simulink library "Thesis_Sublibraries"  (R2020a)
settings: Solver=VariableStepAuto  StartTime=0.0  StopTime=10.0  RelTol=1e-3
undefined symbols (not defined in the file): cga_Horiz_Param, cgb_Horiz_Param, lead_veh_acc, T_mode, Traffic, V2V_FLAG
libraries: simulink x1
settings Model: Creator=John Jr  LastModifiedBy=John Jr
settings SFSimCC: CustomCodeUndefinedFunction=UseInterfaceOnly

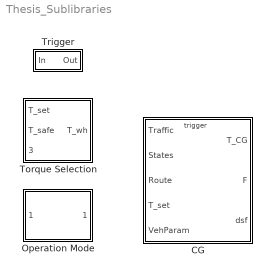
== system Thesis_Sublibraries ==
  CG : Subsystem  TreatAsAtomicUnit=on
      mask Display:
      | patch([0 1 1 0], [0 0 1 1],[.8 1 1])
      | 
      | port_label('input',1,'Traffic')
      | port_label('input',2,'States')
      | port_label('input',3,'Route')
      | port_label('input',4,'T_set')
      | port_label('input',5,'VehParam')
      | 
      | 
      | port_label('output',1,'T_{CG}','texmode','on')
      | port_label('output',2,'F','texmode','on')
      | port_label('output',3,'dsf','texmode','on')
      | 
      | port_label('trigger','\spadesuit','texmode','on')
  Operation Mode : Subsystem  mask{ds_max=200}
      mask prompts: ds_max "Radar Range [m]"
      mask DialogControl Control3 Prompt: Traffic Parameters
      mask Display:
      | patch([0 1 1 0], [0 0 1 1],[.8 1 1])
      | 
      | port_label('input',1,'Traffic')
      | 
      | port_label('output',1,'Mode')
  Torque Selection : Subsystem
      mask Display:
      | patch([0 1 1 0], [0 0 1 1],[.8 1 1])
      | 
      | port_label('input',1,'T_{MPC}','texmode','on')
      | port_label('input',2,'T_{ACC}','texmode','on')
      | port_label('input',3,'Mode')
      | 
      | port_label('output',1,'T_{set}','texmode','on')
  Trigger : Subsystem  mask{f=1}
      mask prompts: f "Trigger Frequency [Hz]"
      mask Display:
      | patch([0 1 1 0], [0 0 1 1],[.8 1 1])
      | 
      | %port_label('input',1,'In')
      | 
      | %port_label('output',1,'Out')
      | 
      | str_f = get_param(gcb,'f');
      | disp(['{\fontname{Cambria Math}f = ' str_f ' Hz}'],'texmode','on')

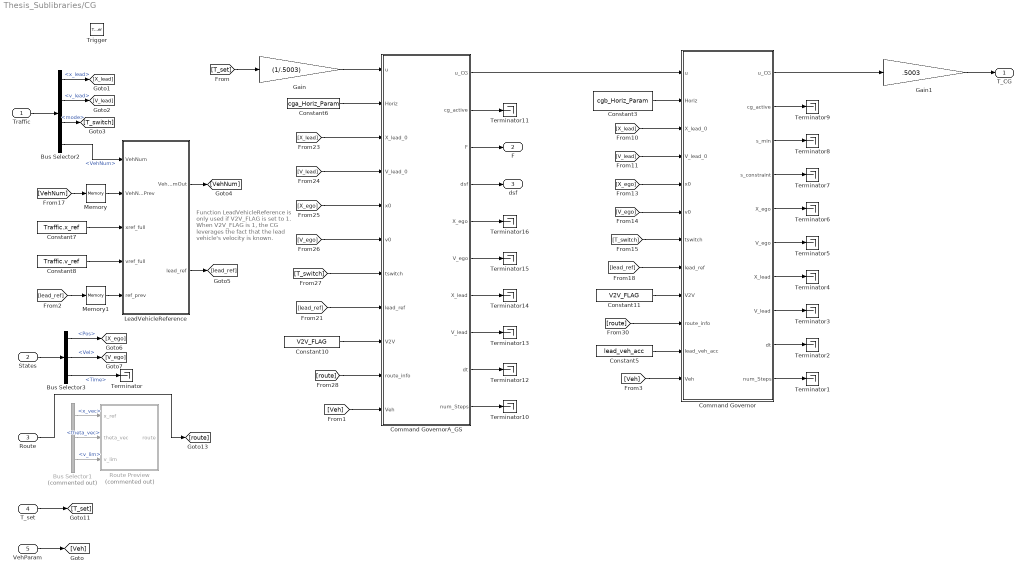
== system Thesis_Sublibraries/CG ==
  note: Function LeadVehicleReference is only used if V2V_FLAG is set to 1. When V2V_FLAG is 1, the CG leverages the fact that the lead vehicle's velocity is known.
  Traffic : Inport
  States : Inport  Port=2
  Route : Inport  Port=3
  T_set : Inport  Port=4
  VehParam : Inport  Port=5
  Trigger : TriggerPort  VariantControl=Variant  PortDimensions=1
  Bus Selector1 : BusSelector  Commented=on  OutputSignals=x_vec,theta_vec,v_lim
  Bus Selector2 : BusSelector  OutputSignals=x_lead,v_lead,mode,VehNum
  Bus Selector3 : BusSelector  OutputSignals=Pos,Vel,Time
  Command Governor : MATLAB Function  TreatAsAtomicUnit=on
  Command GovernorA_GS : MATLAB Function  TreatAsAtomicUnit=on
  Constant10 : Constant  Value=V2V_FLAG
  Constant11 : Constant  Value=V2V_FLAG
  Constant3 : Constant  Value=cgb_Horiz_Param
  Constant5 : Constant  Value=lead_veh_acc
  Constant6 : Constant  Value=cga_Horiz_Param
  Constant7 : Constant  Value=Traffic.x_ref
  Constant8 : Constant  Value=Traffic.v_ref
  Gain : Gain  Gain=(1/.5003)
  Gain1 : Gain  Gain=.5003
  LeadVehicleReference : MATLAB Function  TreatAsAtomicUnit=on
  Memory : Memory  InheritSampleTime=on
  Memory1 : Memory  InheritSampleTime=on
  Route Preview : MATLAB Function  Commented=on  TreatAsAtomicUnit=on
  Terminator{,1..16} (17 alike) : Terminator
  T_CG : Outport  VectorParamsAs1DForOutWhenUnconnected=off
  F : Outport  Port=2  VectorParamsAs1DForOutWhenUnconnected=off
  dsf : Outport  Port=3  VectorParamsAs1DForOutWhenUnconnected=off
  wires:
  Route/1 -> [route]
  Bus Selector3/3 -> Terminator/1  "<Time>"
  Gain1/1 -> T_CG/1
  T_set/1 -> [T_set]
  Bus Selector3/2 -> [V_ego]  "<Vel>"
  Bus Selector3/1 -> [X_ego]  "<Pos>"
  States/1 -> Bus Selector3/1
  Memory/1 -> LeadVehicleReference/2(VehNumPrev)
  [VehNum] -> Memory/1
  Memory1/1 -> LeadVehicleReference/5(ref_prev)
  Constant7/1 -> LeadVehicleReference/3(xref_full)
  LeadVehicleReference/2(lead_ref) -> [lead_ref]
  LeadVehicleReference/1(VehNumOut) -> [VehNum]
  [lead_ref] -> Memory1/1
  Constant8/1 -> LeadVehicleReference/4(vref_full)
  Bus Selector2/4 -> LeadVehicleReference/1(VehNum)  "<VehNum>"
  Bus Selector2/3 -> [T_switch]  "<mode>"
  Bus Selector2/2 -> [V_lead]  "<v_lead>"
  Bus Selector2/1 -> [X_lead]  "<x_lead>"
  Traffic/1 -> Bus Selector2/1
  Bus Selector1/3 -> Route Preview/3(v_lim)  "<v_lim>"
  Bus Selector1/1 -> Route Preview/1(x_ref)  "<x_vec>"
  Bus Selector1/2 -> Route Preview/2(theta_vec)  "<theta_vec>"
  VehParam/1 -> [Veh]
  [T_set] -> Gain/1
  [Veh] -> Command GovernorA_GS/11(Veh)
  Constant11/1 -> Command Governor/9(V2V)
  [Veh] -> Command Governor/12(Veh)
  Command GovernorA_GS/9(dt) -> Terminator12/1
  Command Governor/9(dt) -> Terminator2/1
  [V_lead] -> Command Governor/4(V_lead_0)
  [X_ego] -> Command GovernorA_GS/5(x0)
  [V_ego] -> Command GovernorA_GS/6(v0)
  [T_switch] -> Command Governor/7(tswitch)
  Constant6/1 -> Command GovernorA_GS/2(Horiz)
  Command GovernorA_GS/4(dsf) -> dsf/1
  Command GovernorA_GS/5(X_ego) -> Terminator16/1
  Command GovernorA_GS/1(u_CG) -> Command Governor/1(u)
  [route] -> Command GovernorA_GS/10(route_info)
  Constant10/1 -> Command GovernorA_GS/9(V2V)
  Command Governor/2(cg_active) -> Terminator9/1
  Command Governor/6(V_ego) -> Terminator5/1
  Command GovernorA_GS/2(cg_active) -> Terminator11/1
  [X_lead] -> Command GovernorA_GS/3(X_lead_0)
  [T_switch] -> Command GovernorA_GS/7(tswitch)
  Command GovernorA_GS/7(X_lead) -> Terminator14/1
  Command GovernorA_GS/3(F) -> F/1
  Constant5/1 -> Command Governor/11(lead_veh_acc)
  Command GovernorA_GS/6(V_ego) -> Terminator15/1
  Command Governor/3(s_min) -> Terminator8/1
  [route] -> Command Governor/10(route_info)
  Command GovernorA_GS/10(num_Steps) -> Terminator10/1
  [V_ego] -> Command Governor/6(v0)
  Gain/1 -> Command GovernorA_GS/1(u)
  Command Governor/8(V_lead) -> Terminator3/1
  Command Governor/1(u_CG) -> Gain1/1
  Command Governor/10(num_Steps) -> Terminator1/1
  Constant3/1 -> Command Governor/2(Horiz)
  Command GovernorA_GS/8(V_lead) -> Terminator13/1
  [X_lead] -> Command Governor/3(X_lead_0)
  Command Governor/4(s_constraint) -> Terminator7/1
  Command Governor/7(X_lead) -> Terminator4/1
  [lead_ref] -> Command GovernorA_GS/8(lead_ref)
  Command Governor/5(X_ego) -> Terminator6/1
  [lead_ref] -> Command Governor/8(lead_ref)
  [V_lead] -> Command GovernorA_GS/4(V_lead_0)
  [X_ego] -> Command Governor/5(x0)

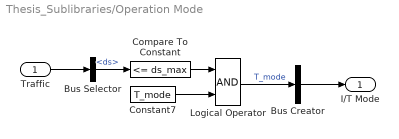
== system Thesis_Sublibraries/Operation Mode ==
  Traffic : Inport
  Bus Creator : BusCreator  Inputs=1
  Bus Selector : BusSelector  OutputSignals=ds
  Compare To Constant : simulink/Logic and Bit Operations/Compare To Constant  relop=<=  const=ds_max  OutDataTypeStr=boolean
  Constant7 : Constant  Value=T_mode
  Logical Operator : Logic  AllPortsSameDT=off  OutDataTypeStr=boolean
  I/T Mode : Outport  VectorParamsAs1DForOutWhenUnconnected=off
  wires:
  Bus Creator/1 -> I/T Mode/1
  Logical Operator/1 -> Bus Creator/1  "T_mode"
  Compare To Constant/1 -> Logical Operator/1
  Bus Selector/1 -> Compare To Constant/1  "<ds>"
  Constant7/1 -> Logical Operator/2
  Traffic/1 -> Bus Selector/1

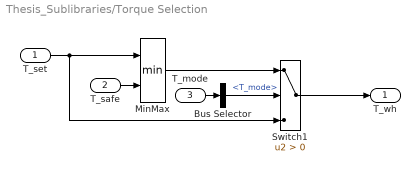
== system Thesis_Sublibraries/Torque Selection ==
  T_set : Inport
  T_safe : Inport  Port=2
  T_mode : Inport  Port=3
  Bus Selector : BusSelector  OutputSignals=T_mode
  MinMax : MinMax  Inputs=2
  Switch1 : Switch  Criteria=u2 > Threshold
  T_wh : Outport  VectorParamsAs1DForOutWhenUnconnected=off
  wires:
  T_safe/1 -> MinMax/2
  T_set/1 -> Switch1/3, MinMax/1
  MinMax/1 -> Switch1/1
  Bus Selector/1 -> Switch1/2  "<T_mode>"
  T_mode/1 -> Bus Selector/1
  Switch1/1 -> T_wh/1

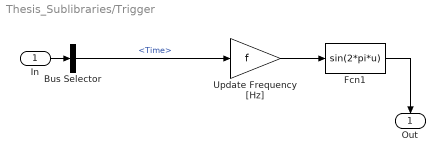
== system Thesis_Sublibraries/Trigger ==
  In : Inport
  Bus Selector : BusSelector  OutputSignals=Time
  Fcn1 : Fcn  Expr=sin(2*pi*u)
  Update Frequency [Hz] : Gain  Gain=f
  Out : Outport  VectorParamsAs1DForOutWhenUnconnected=off
  wires:
  Bus Selector/1 -> Update Frequency [Hz]/1  "<Time>"
  Update Frequency [Hz]/1 -> Fcn1/1
  Fcn1/1 -> Out/1
  In/1 -> Bus Selector/1

== matlab function Thesis_Sublibraries/CG/Command Governor ==
  settings: updateMethod=DISCRETE
  data: u input; u_CG output size=1; Horiz input; X_lead_0 input; V_lead_0 input; cg_active output size=1; x0 input; v0 input; tswitch input; s_min output; lead_ref input size=[8000 3]; s_constraint output; X_ego output; V_ego output; X_lead output; V_lead output; dt output size=1; num_Steps output size=1; V2V input; route_info input; lead_veh_acc input; Veh input
function [u_CG, cg_active, s_min, s_constraint, ...
    X_ego, V_ego, X_lead, V_lead, dt, num_Steps] ... 
    = Command_Governor(u, Horiz, X_lead_0, ... 
        V_lead_0, x0, v0, tswitch,...
        lead_ref, V2V, route_info, lead_veh_acc, Veh)
% s_constraint = NaN(1, 80);
s_constraint    = NaN(1, length(Horiz));
X_ego           = zeros(1, length(Horiz));
V_ego           = zeros(1, length(Horiz));
X_lead          = zeros(1, length(Horiz));
V_lead          = V_lead_0.*ones(1, length(Horiz));
Cs_min          = 10;


cg_Step         = Horiz(1);
% num_Steps       = cg_length/cg_Step;
num_Steps       = length(Horiz);
dt              = cg_Step;
u_brk_max       = -120000;

xref = lead_ref(:,1);
vref = lead_ref(:,2);
tref = lead_ref(:,3);

tsafe = 1;

X_vec = route_info(:,1);                                %   rad - Road grade angle vector
theta_vec = route_info(:,2);                            %   rad - Road grade angle vector


amdego          = -3;  
percBuff        = 1;
X_ego(1)        = x0;
V_ego(1)        = v0;
X_lead(1)       = X_lead_0;
d_u             = 200;

t_cg = zeros(1, length(Horiz)+1);
t_cg(2:end) = cumsum(Horiz);

if tswitch ~= 1
    u_CG = u;
    cg_active = 0;
    s_min = nan;
    MAX_FLAG = 0;
else
    if V2V == 1
        t_shift = interpone(xref, tref, X_lead_0);
        
        for i = 2:length(Horiz)
            X_lead(i) = interpone(tref, xref, t_shift + t_cg(i));
            V_lead(i) = interpone(xref, vref, X_lead(i));
        end
    else
        for i = 2:length(Horiz)
            V_lead(i) = V_lead(i-1) + lead_veh_acc*dt;
            X_lead(i) = X_lead(i-1) + ((V_lead(i) + V_lead(i-1))/2)*dt;
        end
    end
    
    
%     amdlead = a_lead_brk_max;
%     i = 1;
%     tstoplead = abs(V_lead(i)/a_lead_brk_max);
%     
%     if a_lead_brk_max == 0
%         s_min = Cs_min;
%     else
%         tstopego = abs(V_ego(i)/amdego);
%         s_min = max(Cs_min, Cs_min + (V_ego(i)*tstopego - V_lead(i)*tstoplead) ...
%                 + ((amdego/2)*tstopego^2 - (amdlead/2)*tstoplead^2));
% 
%     end
    s_min = max(Cs_min, tsafe*V_lead(1));
    
    MAX_FLAG = 0;
    u_CG = u;
    i = 1;
    while i < num_Steps && MAX_FLAG == 0
        
        % Veh(1)    g
        % Veh(2)    rho
        % Veh(3)    m
        % Veh(4)    Cd
        % Veh(5)    A_ref
        % Veh(6)    Cr
        theta = interp1(X_vec, theta_vec, X_ego(i));
        F_grav = Veh(3)*Veh(1)*sin(theta);
        F_road = Veh(3)*Veh(1)*Veh(6)*cos(theta);
        F_aero = (1/2)*Veh(4)*Veh(2)*Veh(5)*V_ego(i)^2;
        V_ego(i+1) = V_ego(i) + (dt/Veh(3))*(u_CG) - percBuff*(dt/Veh(3))*(F_road + F_aero ...
            + max(0, F_grav)) - (dt/Veh(3))*min(0, F_grav)*(1+(1-percBuff));
        X_ego(i+1) = X_ego(i) + ((V_ego(i) + V_ego(i+1))/2)*dt;  
       
        s = X_lead(i) - X_ego(i);
        
%         rho = V_ego(i) - V_lead(i);
%         tstopego = abs(V_ego(i)/amdego);
%         tstoplead = abs(V_lead(i)/a_lead_brk_max);
%         if a_lead_brk_max == 0
%             s_constraint(i) = Cs_min;
%         else
%             
%             s_constraint(i) = max(Cs_min, Cs_min + (V_ego(i)*tstopego ...
%                 - V_lead(i)*tstoplead) ... 
%                 + ((amdego/2)*tstopego^2 - (amdlead/2)*tstoplead^2));
%         end
        s_constraint(i) = max(Cs_min, tsafe*V_lead(i));
        
        if i == 1
            s_min = s_constraint(i);
        end
        if i == 1 && s < s_constraint(i)
            u_CG = u_brk_max;
            MAX_FLAG = 1;
            s_min = s_constraint(i);
        else
            if s < s_constraint(i)
                i = 1;
                if u_CG - d_u < u_brk_max
                    MAX_FLAG = 1;
                else
                    u_CG = u_CG - d_u;
                end
            else
                i = i+1;
            end
        end
    end
    if u_CG ~= u
        cg_active = 1; 
    else
        cg_active = 0;
    end
end


function return_val = interpone(X_data, Y_data, X_q)
    if X_q >= X_data(1) && X_q <= X_data(end)
        [~, I] = min((X_q - X_data).^2);
        if X_data(I) > X_q
            x_ub = X_data(I);
            x_lb = X_data(I-1);
            ind_xub = I;
            ind_xlb = I-1;
        else
            x_lb = X_data(I);
            ind_xlb = I;
            if I+1 >= length(X_data)    % M is probably equal to X_q and also the max value 
                x_lb = X_data(I-1);
                x_ub = I;
                ind_xub = I;
                ind_xlb = I-1;
            else
                x_ub = X_data(I+1);
                ind_xub = I+1;
            end
        end 
        y_0 = Y_data(ind_xlb);
        y_1 = Y_data(ind_xub);
        return_val = y_0 + (X_q - x_lb)*((y_1 - y_0)/(x_ub - x_lb));  
    else
        return_val = 3.141; %debug help
    end
end


end

== matlab function Thesis_Sublibraries/CG/Command GovernorA_GS ==
  data: u input; u_CG output size=1; Horiz input; X_lead_0 input; V_lead_0 input; cg_active output size=1; x0 input; v0 input; tswitch input; F output; dsf output; X_ego output; lead_ref input size=[8000 3]; V_ego output; X_lead output; V_lead output; dt output; num_Steps output; V2V input; route_info input; Veh input
function [u_CG, cg_active, F, dsf, X_ego, V_ego, X_lead, ... 
    V_lead, dt, num_Steps] = Command_GovernorA_GS(u, Horiz, X_lead_0, ... 
        V_lead_0, x0, v0, tswitch, lead_ref, V2V, route_info, Veh)

% Cs_min = 10;
% X_lead_0        = vehicle(1);   % Lead vehicle position [m]
% V_lead_0        = vehicle(2);   % Lead vehicle velocity [m/s]
% x0              = vehicle(3);   % Ego vehicle position [m]
% v0              = vehicle(4);   % Ego vehicle velocity [m/s]
large_headway    = 2;
% rho_a           = 1.2;
% Cd              = 0.49;
% A_ref           = 10.67;
% m               = 35000;
% g               = 9.81;
% Cr              = 0.00551;
% k_D             = .5*Cd*rho_a*A_ref;
% cg_length       = sum(Horiz);
cg_Step         = Horiz(1);
% num_Steps       = cg_length/cg_Step;
num_Steps       = length(Horiz);
dt              = cg_Step;
u_brk_max       = -120000;
% amdego          = -3;
xref = lead_ref(:,1);
vref = lead_ref(:,2);
tref = lead_ref(:,3);

X_vec = route_info(:,1);                                %   rad - Road grade angle vector
theta_vec = route_info(:,2);                            %   rad - Road grade angle vector

X_ego           = zeros(1, num_Steps+1);
V_ego           = zeros(1, num_Steps+1);
X_ego(1)        = x0;
V_ego(1)        = v0;
X_lead          = zeros(1, num_Steps);
X_lead(1)       = X_lead_0;
V_lead          = V_lead_0.*ones(1, num_Steps);

t_cg = zeros(1, length(Horiz)+1);
t_cg(2:end) = cumsum(Horiz);

du = 50;
if tswitch ~= 1
    u_CG = u;
    cg_active = 0;
    
    F = 255;
    dsf = 255;
else
    if V2V == 1
        t_shift = interpone(xref, tref, X_lead_0);
        
        for i = 2:length(Horiz)
            X_lead(i) = interpone(tref, xref, t_shift + t_cg(i));
            V_lead(i) = interpone(xref, vref, X_lead(i));
        end
    else
        for i = 2:length(Horiz)
            X_lead(i) = X_lead(i-1) + ((V_lead(i) + V_lead(i-1))/2)*dt;
        end
    end
    
    X_des_fin = X_lead(end) - large_headway*V_lead(end);
    
    F_0 = objFunc(u, X_des_fin, X_ego, V_ego, num_Steps, dt, u, X_vec, theta_vec, Veh);
    if F_0 == 0
        u_CG = u;
        [F, dsf] = objFunc2(u_CG, X_des_fin, X_ego, V_ego, num_Steps, dt, u, X_vec, theta_vec, Veh);
    else
        objF = @(u_var) objFunc(u_var, X_des_fin, X_ego, V_ego, num_Steps, dt, u, X_vec, theta_vec, Veh);
        stepsize = 100; %N
        [xleft, xright] = hw2p2BoundingPhaseAlg(u, stepsize, objF);
        conv = 0.2;
        [~, ~, ~, ~, xopt, ~, ~, ~, ~, ~] = goldenSection(xleft, xright, conv, objF);
        %         index = sum(~isnan(xopt));
        %         u_opt = xopt(index);
        u_CG = max(u_brk_max, xopt);
        [F, dsf] = objFunc2(u_CG, X_des_fin, X_ego, V_ego, num_Steps, dt, u, X_vec, theta_vec, Veh);
    end
    
    
    
    if u_CG ~= u
        cg_active = 1;
    else
        cg_active = 0;
    end
end

end
%%
function [xleft, xright] = hw2p2BoundingPhaseAlg(x0, stepsize, objF)
    FLAG = 0;
    count = 0;
    x_prev = x0;            %line isnecessary to generate c code
    x_prev2 = x0;           %line isnecessary to generate c code
    delta = abs(stepsize);  %line isnecessary to generate c code
    F_0   = objF(x0);       %line isnecessary to generate c code
    F_prev = F_0;           %line isnecessary to generate c code
    xleft = x0;             %line isnecessary to generate c code
    xright = x0;            %line isnecessary to generate c code
    while FLAG == 0 && count < 100
       %% first iteration through, must calculate delta
       if count == 0
           F_dec = objF(x0 - abs(stepsize));
           F_inc = objF(x0 + abs(stepsize));
           if F_dec >= F_0 && F_0 >= F_inc
               delta = abs(stepsize);
           elseif F_dec <= F_0 && F_0 <= F_inc
               delta = -abs(stepsize);
           else
%                if F_inc > F_dec
                    xright = x0 + abs(stepsize);
                    xleft  = x0 - abs(stepsize);
                    FLAG = 1;
%                else
%                     xright = x0 - abs(stepsize);
%                     xleft  = x0 + abs(stepsize);
%                end
           end
       end
       %% rest
       if FLAG == 0
           x_next = x_prev + (2^count)*(delta);
           F_next = objF(x_next);
           if F_next < F_prev
               F_prev = F_next;
               x_prev2 = x_prev;
               x_prev = x_next;
               count = count + 1;
           else
               xleft = x_prev2;
               xright = x_next;
               %            x_prev = x_prev2;  %pointless line necessary to generate c code
               FLAG = 1;
           end
       end
       
    end

end
%%
function [xl, x1, x2, xr, xopt, fl, f1, f2, fr, fopt] = goldenSection(xleft, xright, conv, objF)
L_orig = xright-xleft;
x = zeros(1,4); x(1) = xleft; x(4) = xright;
FLAG = 0;
count = 0;
% % % % % x1 = 0; xl = 0;
xl      = 0;
x1      = 0;
x2      = 0;
xr      = 0;
L       = 0;
fl      = 0;
f1      = 0;
f2      = 0;
fr      = 0;
xopt    = 0;
fopt    = 0;
while FLAG == 0 && count <10000
    count = count + 1;
    xl = x(1); x1 = x(2); x2 = x(3); xr = x(4);
    L = x(4) - x(1);
    gamma = 0.618;
    x(2) = x(1) + (1-gamma)*L; x(3) = x(4) - (1-gamma)*L;
    
    f_2 = objF(x(2));
    f_3 = objF(x(3));
    
    fl = objF(x(1)); f1 = f_2; 
    f2 = f_3; fr = objF(x(4));
    if f_3 > f_2
        x_opt = (x(2)+x(3))/2;
        f_opt = objF(x_opt);
         x(4) = x(3);
    else
        x_opt = (x(2)+x(3))/2;
        f_opt = objF(x_opt);
        x(1) = x(2);
    end
    xopt = x_opt;
    fopt = f_opt;
    Lnew = x(4) - x(1);
    if Lnew/L_orig < conv
        FLAG = 1;
        fopt = objF(x_opt);
    end
%     x_range = [x(1) x(4)];
end

end
%%

function F = objFunc(u, X_des_fin, X_ego, V_ego, num_Steps, dt, u_0, X_vec, theta_vec, Veh)
% Veh(1)    g
% Veh(2)    rho 
% Veh(3)    m 
% Veh(4)    Cd 
% Veh(5)    A_ref 
% Veh(6)    Cr 
% Veh(7)    r_wheel 
% Veh(8)    J_wheel 
% Veh(9)    EV_J 
% Veh(10)   fgr.rt 

for i = 1:num_Steps
% %     theta = interpone(X_vec, theta_vec, X_ego(i), 'str', 0);
%     V_ego(i+1) = V_ego(i) + (dt/35000)*(u) - (dt/35000)*(35000*9.81*0.00551 + 0.5*0.49*1.2*10.67*V_ego(i)^2);
%     X_ego(i+1) = X_ego(i) + ((V_ego(i) + V_ego(i+1))/2)*dt;
    theta = interp1(X_vec, theta_vec, X_ego(i));
    F_grav = Veh(3)*Veh(1)*sin(theta);
    F_road = Veh(3)*Veh(1)*Veh(6)*cos(theta);
    F_aero = (1/2)*Veh(4)*Veh(2)*Veh(5)*V_ego(i)^2;
    V_ego(i+1) = V_ego(i) + (dt/Veh(3))*(u) - (dt/Veh(3))*(F_road + F_aero ...
        + F_grav);
    X_ego(i+1) = X_ego(i) + ((V_ego(i) + V_ego(i+1))/2)*dt;
end

if max(min(0, X_des_fin - X_ego(end))) == 0
    F = (u - u_0).^2;
else
    F = (X_des_fin - X_ego(end)).^2;
end

end

function return_val = interpone(X_data, Y_data, X_q)
    if X_q >= X_data(1) && X_q <= X_data(end)
        [~, I] = min((X_q - X_data).^2);
        if X_data(I) > X_q
            x_ub = X_data(I);
            x_lb = X_data(I-1);
            ind_xub = I;
            ind_xlb = I-1;
        else
            x_lb = X_data(I);
            ind_xlb = I;
            if I+1 >= length(X_data)    % M is probably equal to X_q and also the max value 
                x_lb = X_data(I-1);
                x_ub = I;
                ind_xub = I;
                ind_xlb = I-1;
            else
                x_ub = X_data(I+1);
                ind_xub = I+1;
            end
        end 
        y_0 = Y_data(ind_xlb);
        y_1 = Y_data(ind_xub);
        return_val = y_0 + (X_q - x_lb)*((y_1 - y_0)/(x_ub - x_lb));  
    else
        return_val = 3.141; %debug help
    end
end

function [F, dsf] = objFunc2(u, X_des_fin, X_ego, V_ego, num_Steps, dt, u_0, X_vec, theta_vec, Veh)
% Veh(1)    g
% Veh(2)    rho 
% Veh(3)    m 
% Veh(4)    Cd 
% Veh(5)    A_ref 
% Veh(6)    Cr 
% Veh(7)    r_wheel 
% Veh(8)    J_wheel 
% Veh(9)    EV_J 
% Veh(10)   fgr.rt 

for i = 1:num_Steps
    %     theta = interpone(X_vec, theta_vec, X_ego(i), 'str', 0);
    theta = interp1(X_vec, theta_vec, X_ego(i));
    F_grav = Veh(3)*Veh(1)*sin(theta);
    F_road = Veh(3)*Veh(1)*Veh(6)*cos(theta);
    F_aero = (1/2)*Veh(4)*Veh(2)*Veh(5)*V_ego(i)^2;
    V_ego(i+1) = V_ego(i) + (dt/Veh(3))*(u) - (dt/Veh(3))*(F_road + F_aero ...
        + F_grav);
    X_ego(i+1) = X_ego(i) + ((V_ego(i) + V_ego(i+1))/2)*dt;
end
dsf = X_des_fin-X_ego(end);
if max(min(0, X_des_fin - X_ego(end))) == 0
    F = (u - u_0).^2;
else
    F = (X_des_fin - X_ego(end)).^2;
end

end

== matlab function Thesis_Sublibraries/CG/Route Preview ==
  data: x_ref input; route output size=[2000,3]; theta_vec input; v_lim input
function route = fcn(x_ref,theta_vec,v_lim)

route = [x_ref,theta_vec,v_lim];

== matlab function Thesis_Sublibraries/CG/LeadVehicleReference ==
  data: VehNum input; VehNumOut output; VehNumPrev input; xref_full input; vref_full input; lead_ref output; ref_prev input
function [VehNumOut, lead_ref] = LeadVehicleReference(VehNum, VehNumPrev, xref_full, vref_full, ...
    ref_prev)

xref_prev = ref_prev(:, 1);
vref_prev = ref_prev(:, 2);
tref_prev = ref_prev(:, 3);


VehNumOut = VehNum;
if VehNum == VehNumPrev
    if VehNum == 0
        xref = zeros(length(xref_full(:, 1)), 1);
        vref = zeros(length(xref_full(:, 1)), 1);
        tref = zeros(length(xref_full(:, 1)), 1);
        
        lead_ref = [xref vref tref];
    else
        tref = tref_prev;
        xref = xref_prev;
        vref = vref_prev;
        lead_ref = [xref vref tref];
    end
else
    tref = zeros(length(xref_full(:, 1)), 1);
    xref = xref_full(:, VehNum);
    vref = vref_full(:, VehNum);
    for i = 2:length(xref)
        ds      = xref(i) - xref(i-1);
        vmean   = mean([vref(i) vref(i-1)]);
        tref(i) = ds/vmean;
    end
    tref = cumsum(tref);
    lead_ref = [xref vref tref];
end
